simulink model "MyTestModel"  (R2019a)
settings: Solver=FixedStepDiscrete  StartTime=0.0  StopTime=10.0  FixedStep=TSamp  RelTol=1e-3
values from neighbouring files (symbols this model uses):
  maxValue = Simulink.Parameter    [initModel.m]
  TSamp = 0.1    [initModel.m]
settings Model: Creator=lrosqvis  LastModifiedBy=mluo
settings DataIOCC: SaveOutput=off  SaveTime=off
settings OptimizationCC: DefaultParameterBehavior=Inlined  UseDivisionForNetSlopeComputation=on  InlineInvariantSignals=on  PassReuseOutputArgsAs=Individual arguments  EfficientFloat2IntCast=on  LifeSpan=Inf
settings DebuggingCC: ReadBeforeWriteMsg=DisableAll  WriteAfterWriteMsg=DisableAll  WriteAfterReadMsg=DisableAll  AlgebraicLoopMsg=error  ArtificialAlgebraicLoopMsg=error  SaveWithDisabledLinksMsg=error  SaveWithParameterizedLinksMsg=error  BlockPriorityViolationMsg=error  SolverPrmCheckMsg=error  InheritedTsInSrcMsg=error  MultiTaskDSMMsg=none  SingleTaskRateTransMsg=error  TasksWithSamePriorityMsg=error  SigSpecEnsureSampleTimeMsg=error  IntegerOverflowMsg=error  ParameterUnderflowMsg=error  ParameterPrecisionLossMsg=error  ParameterTunabilityLossMsg=error  UnderSpecifiedDataTypeMsg=error  UnnecessaryDatatypeConvMsg=warning  VectorMatrixConversionMsg=error  SignalLabelMismatchMsg=error  UnconnectedInputMsg=error  UnconnectedOutputMsg=error  UnconnectedLineMsg=error  SFcnCompatibilityMsg=error  BusObjectLabelMismatch=error  RootOutportRequireBusObject=error  AssertControl=DisableAll  ModelReferenceIOMsg=error  ModelReferenceIOMismatchMessage=error  UnknownTsInhSupMsg=error  ModelReferenceDataLoggingMessage=error  StateNameClashWarn=warning  PregeneratedLibrarySubsystemCodeDiagnostic=none  StrictBusMsg=ErrorOnBusTreatedAsVector  NonBusSignalsTreatedAsBus=error  SFInvalidInputDataAccessInChartInitDiag=error  SFTransitionOutsideNaturalParentDiag=error  SFUnreachableExecutionPathDiag=error  SFUndirectedBroadcastEventsDiag=error  SFTransitionActionBeforeConditionDiag=error  IntegerSaturationMsg=error  ArithmeticOperatorsInVariantConditions=warning
settings ModelReferenceCC: UpdateModelReferenceTargets=IfOutOfDate
settings SFSimCC: SFSimEcho=off  SimUseLocalCustomCode=off  CompileTimeRecursionLimit=0  EnableRuntimeRecursion=off  MATLABDynamicMemAlloc=off
settings RTWCC: SystemTargetFile=ert.tlc  GenCodeOnly=on  TemplateMakefile=ert_default_tmf  GenerateReport=on  RTWUseLocalCustomCode=off  BuildConfiguration=Faster Runs  IncludeHyperlinkInReport=on  PortableWordSizes=on  GenerateTraceInfo=on
settings CodeAppCC: ForceParamTrailComments=on  IgnoreCustomStorageClasses=off  IgnoreTestpoints=on  OperatorAnnotations=on  SimulinkDataObjDesc=on  SFDataObjDesc=on  MATLABFcnDesc=on  MangleLength=4  InsertBlockDesc=on  InsertPolySpaceComments=on  StateflowObjectComments=on  MATLABSourceComments=on  ReqsInCode=on
settings ERTTargetCC: TargetLangStandard=C99 (ISO)  UtilityFuncGeneration=Shared location  GenerateSampleERTMain=on  IncludeMdlTerminateFcn=off  SuppressErrorStatus=on  SupportAbsoluteTime=off  SupportNonFinite=off  ParenthesesLevel=Maximum  CastingMode=Standards  GenerateSharedConstants=off  InlinedParameterPlacement=NonHierarchical  ERTCustomFileTemplate=example_file_process.tlc  PreserveExpressionOrder=on  PreserveIfCondition=on  EnableSignedLeftShifts=off  EnableSignedRightShifts=off
settings ConfigComp: CovEnable=on  RecordCoverage=on  CovMetricSettings=dcwe  CovModelRefEnable=on  PSAutoStubLUT=on

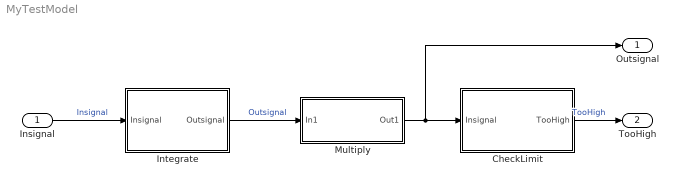
== system MyTestModel ==
  Insignal : Inport  OutDataTypeStr=double  PortDimensions=1  SampleTime=TSamp
  CheckLimit : Subsystem
  Integrate : Subsystem
  Multiply : Subsystem
  Outsignal : Outport  OutDataTypeStr=double  PortDimensions=1  SampleTime=TSamp
  TooHigh : Outport  Port=2  OutDataTypeStr=boolean  PortDimensions=1  SampleTime=TSamp
  wires:
  Insignal/1 -> Integrate/1(Insignal)  "Insignal"
  CheckLimit/1(TooHigh) -> TooHigh/1  "TooHigh"
  Integrate/1(Outsignal) -> Multiply/1(In1)  "Outsignal"
  Multiply/1(Out1) -> CheckLimit/1(Insignal), Outsignal/1

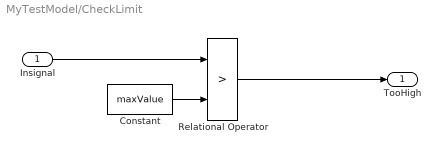
== system MyTestModel/CheckLimit ==
  Insignal : Inport
  Constant : Constant  Value=maxValue
  Relational Operator : RelationalOperator  Operator=>  OutDataTypeStr=boolean  RndMeth=Nearest
  TooHigh : Outport
  wires:
  Relational Operator/1 -> TooHigh/1
  Insignal/1 -> Relational Operator/1
  Constant/1 -> Relational Operator/2

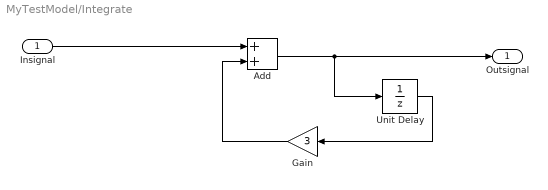
== system MyTestModel/Integrate ==
  Insignal : Inport
  Add : Sum
  Gain : Gain  Gain=3
  Unit Delay : UnitDelay  SampleTime=-1  HasFrameUpgradeWarning=on
  Outsignal : Outport
  wires:
  Insignal/1 -> Add/1
  Add/1 -> Outsignal/1, Unit Delay/1
  Unit Delay/1 -> Gain/1
  Gain/1 -> Add/2

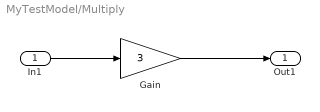
== system MyTestModel/Multiply ==
  In1 : Inport
  Gain : Gain  Gain=3
  Out1 : Outport
  wires:
  In1/1 -> Gain/1
  Gain/1 -> Out1/1
